simulink library "speedgoatlib_evse"  (R2024b)
settings: Solver=VariableStepAuto  StartTime=0.0  StopTime=10.0  RelTol=1e-3
undefined symbols (not defined in the file): sg_ev_charging_read_m, sg_ev_charging_write_m, sg_ev_isolation_read_m, sg_ev_parameter_read_m, sg_ev_parameter_write_m, sg_ev_precharge_read_m, sg_ev_precharge_write_m, sg_ev_status_m, sg_ev_stop_read_m, sg_ev_stop_write_m, sg_ev_welding_read_m, sg_ev_welding_write_m, sg_evse_charging_read_m, sg_evse_charging_write_m, sg_evse_isolation_read_m, sg_evse_isolation_write_m, sg_evse_parameter_read_m, sg_evse_parameter_write_m, sg_evse_precharge_read_m, sg_evse_precharge_write_m, sg_evse_status_m, sg_evse_stop_read_m, sg_evse_stop_write_m, sg_evse_welding_read_m, sg_evse_welding_write_m
libraries: speedgoatlib_mqtt x199, simulink x39, $bdroot x24
(part 7 of 8)

== system speedgoatlib_evse/Blocks by Charge State/EVSE Welding Read /Enabled Subsystem ==
  Enable : EnablePort
  ASCII to String : ASCIIToString
  ASCII to String1 : ASCIIToString
  ASCII to String2 : ASCIIToString
  Data Type Conversion1 : DataTypeConversion  OutDataTypeStr=boolean  SaturateOnIntegerOverflow=off  RndMeth=Floor
  String to Double : ScanString  Format="\"%lf\""
  String to Double1 : ScanString  Format="\"%lf\""
  String to Double2 : ScanString  Format="\"%lf\""
  port0_ci_ev_welding_errorcode : S-Function  FunctionName=sg_mqtt_client_subscribe_s  Parameters="ClientId,  ConnectionId, Topic, QoS, InitValue, Extended, SampleTime"  SFunctionDeploymentMode=off  EnableBusSupport=off  mask(mqtt_client_subscribe_1){ClientId=parClientId, ConnectionId=parConnectionId, Topic='port0/ci/ev/welding/errorcode', QoS=0 - at most once, InitValue=zeros(1,24,'uint8'), Extended=off, SampleTime=parSampleTime}
      mask prompts: ClientId "Station ID"; ConnectionId "Connection ID"; QoS "Quality of Service"; InitValue "Init Value"; Extended "Extended Interface"; SampleTime "Sample Time [s]"
      mask help: Speedgoat Driver Block<br>MQTT Client - Subscribe<br><br>&copy; 2007 - 2023, Speedgoat GmbH, <a href="matlab: web('www.speedgoat.com','-browser');">www.speedgoat.com</a>
      mask init:
      | sg_mqtt_client_subscribe_m.runMaskInitialization(ClientId, ConnectionId, Topic, InitValue, Extended);
      mask Help: eval('sg.utils.help.show(''io_main/refentry_mqtt_client_subscribe'');')
      mask TypeOptions QoS: 0 - at most once | 1 - at least once | 2 - exactly once
      mask DialogControl groupParameters Prompt: Parameters
      mask Display: disp('Speedgoat\nMQTT Client\nSubscribe\nStation ID: 0\nConnection ID: 0');
  port0_ci_ev_welding_ready : speedgoatlib_mqtt/Client/MQTT Client Subscribe  ClientId=parClientId  ConnectionId=parConnectionId  Topic='port0/ci/ev/welding/ready'  QoS=0 - at most once  InitValue=zeros(1,12,'uint8')  Extended=off  SampleTime=parSampleTime
      settings: SourceProductName=MQTT
  port0_ci_ev_welding_resssoc : S-Function  FunctionName=sg_mqtt_client_subscribe_s  Parameters="ClientId,  ConnectionId, Topic, QoS, InitValue, Extended, SampleTime"  SFunctionDeploymentMode=off  EnableBusSupport=off  mask(mqtt_client_subscribe_1){ClientId=parClientId, ConnectionId=parConnectionId, Topic='port0/ci/ev/welding/resssoc', QoS=0 - at most once, InitValue=zeros(1,12,'uint8'), Extended=off, SampleTime=parSampleTime}
      mask prompts: ClientId "Station ID"; ConnectionId "Connection ID"; QoS "Quality of Service"; InitValue "Init Value"; Extended "Extended Interface"; SampleTime "Sample Time [s]"
      mask help: Speedgoat Driver Block<br>MQTT Client - Subscribe<br><br>&copy; 2007 - 2023, Speedgoat GmbH, <a href="matlab: web('www.speedgoat.com','-browser');">www.speedgoat.com</a>
      mask init:
      | sg_mqtt_client_subscribe_m.runMaskInitialization(ClientId, ConnectionId, Topic, InitValue, Extended);
      mask Help: eval('sg.utils.help.show(''io_main/refentry_mqtt_client_subscribe'');')
      mask TypeOptions QoS: 0 - at most once | 1 - at least once | 2 - exactly once
      mask DialogControl groupParameters Prompt: Parameters
      mask Display: disp('Speedgoat\nMQTT Client\nSubscribe\nStation ID: 0\nConnection ID: 0');
  EV Ready : Outport
  EV Errorcode : Outport  Port=2
  EV RESS SOC : Outport  Port=3
  wires:
  Data Type Conversion1/1 -> EV Ready/1
  port0_ci_ev_welding_resssoc/1 -> ASCII to String2/1
  ASCII to String2/1 -> String to Double2/1
  String to Double2/1 -> EV RESS SOC/1
  String to Double1/1 -> EV Errorcode/1
  String to Double/1 -> Data Type Conversion1/1
  ASCII to String1/1 -> String to Double/1
  ASCII to String/1 -> String to Double1/1
  port0_ci_ev_welding_errorcode/1 -> ASCII to String/1
  port0_ci_ev_welding_ready/1 -> ASCII to String1/1

== system speedgoatlib_evse/Blocks by Charge State/EVSE Welding Read /string compare logic ==
  Input : Inport
  ASCII to String1 : ASCIIToString
  Add : Sum
  Gain : Gain  Gain=2
  String Compare : StringCompare
  String Compare1 : StringCompare
  String Constant : StringConstant  String="\"started\""
  String Constant1 : StringConstant  String="\"finished\""
  Out1 : Outport
  wires:
  ASCII to String1/1 -> String Compare1/1, String Compare/1
  String Constant1/1 -> String Compare1/2
  String Compare/1 -> Add/1
  String Constant/1 -> String Compare/2
  String Compare1/1 -> Gain/1
  Gain/1 -> Add/2
  Add/1 -> Out1/1
  Input/1 -> ASCII to String1/1

== system speedgoatlib_evse/Blocks by Charge State/EVSE Welding Write /Enabled Subsystem ==
  notification : Inport
  isolationstatus : Inport  Port=2
  statuscode : Inport  Port=3
  presentvoltage : Inport  Port=4
  Enable : EnablePort
  Constant1 : Constant  Value=parEnIsolationStatus  OutDataTypeStr=boolean
  Constant2 : Constant  Value=parEnStatusCode  OutDataTypeStr=boolean
  Constant3 : Constant  Value=parEnPresentVoltage  OutDataTypeStr=boolean
  Constant8 : Constant  Value=parEnNotification  OutDataTypeStr=boolean
  Data Type Conversion3 : DataTypeConversion  OutDataTypeStr=double  SaturateOnIntegerOverflow=off  RndMeth=Floor
  Data Type Conversion4 : DataTypeConversion  OutDataTypeStr=double  SaturateOnIntegerOverflow=off  RndMeth=Floor
  Function Caller11 : FunctionCaller  FunctionPrototype=json_string = toJsonPhysicalValue(multiplier,value)  InputArgumentSpecifications=double(0), double(0)  OutputArgumentSpecifications=zeros(1,48,'uint8')
  Ground{1..3,8} (4 alike) : Ground
  Simulink Function2 : Subsystem  TreatAsAtomicUnit=on
  String to ASCII1 : StringToASCII  OutputVectorSize=12
  String to ASCII2 : StringToASCII  OutputVectorSize=12
  String to ASCII3 : StringToASCII  OutputVectorSize=16
  To String1 : ToString
  To String2 : ToString
  To String3 : ToString
  port0_ci_evse_welding_isolationstatus : speedgoatlib_mqtt/Client/MQTT Client Publish  ClientId=parClientId  ConnectionId=parConnectionId  Topic='port0/ci/evse/welding/isolationstatus'  QoS=0 - at most once  Retain=on  Extended=on  SampleTime=parSampleTime
      settings: SourceProductName=MQTT
  port0_ci_evse_welding_notification : speedgoatlib_mqtt/Client/MQTT Client Publish  ClientId=parClientId  ConnectionId=parConnectionId  Topic='port0/ci/evse/welding/notification'  QoS=0 - at most once  Retain=on  Extended=on  SampleTime=parSampleTime
      settings: SourceProductName=MQTT
  port0_ci_evse_welding_presentvoltage : speedgoatlib_mqtt/Client/MQTT Client Publish  ClientId=parClientId  ConnectionId=parConnectionId  Topic='port0/ci/evse/welding/presentvoltage'  QoS=0 - at most once  Retain=on  Extended=on  SampleTime=parSampleTime
      settings: SourceProductName=MQTT
  port0_ci_evse_welding_statuscode : speedgoatlib_mqtt/Client/MQTT Client Publish  ClientId=parClientId  ConnectionId=parConnectionId  Topic='port0/ci/evse/welding/statuscode'  QoS=0 - at most once  Retain=on  Extended=on  SampleTime=parSampleTime
      settings: SourceProductName=MQTT
  to physical value format : MATLAB Function  TreatAsAtomicUnit=on
  wires:
  presentvoltage/1 -> to physical value format/1(input)
  Function Caller11/1 -> port0_ci_evse_welding_presentvoltage/1
  to physical value format/1(multiplier) -> Function Caller11/1
  to physical value format/2(value) -> Function Caller11/2
  Ground8/1 -> port0_ci_evse_welding_notification/3
  To String3/1 -> String to ASCII3/1
  Constant8/1 -> port0_ci_evse_welding_notification/2
  String to ASCII3/1 -> port0_ci_evse_welding_notification/1
  notification/1 -> To String3/1
  To String1/1 -> String to ASCII1/1
  String to ASCII1/1 -> port0_ci_evse_welding_isolationstatus/1
  Data Type Conversion3/1 -> To String1/1
  isolationstatus/1 -> Data Type Conversion3/1
  To String2/1 -> String to ASCII2/1
  statuscode/1 -> Data Type Conversion4/1
  String to ASCII2/1 -> port0_ci_evse_welding_statuscode/1
  Data Type Conversion4/1 -> To String2/1
  Constant1/1 -> port0_ci_evse_welding_isolationstatus/2
  Ground1/1 -> port0_ci_evse_welding_isolationstatus/3
  Ground2/1 -> port0_ci_evse_welding_statuscode/3
  Constant2/1 -> port0_ci_evse_welding_statuscode/2
  Constant3/1 -> port0_ci_evse_welding_presentvoltage/2
  Ground3/1 -> port0_ci_evse_welding_presentvoltage/3

== system speedgoatlib_evse/Blocks by Charge State/EVSE Welding Write /string compare logic ==
  Input : Inport
  ASCII to String1 : ASCIIToString
  Add : Sum
  Gain : Gain  Gain=2
  String Compare : StringCompare
  String Compare1 : StringCompare
  String Constant : StringConstant  String="\"started\""
  String Constant1 : StringConstant  String="\"finished\""
  Out1 : Outport
  wires:
  Input/1 -> ASCII to String1/1
  Add/1 -> Out1/1
  Gain/1 -> Add/2
  String Compare1/1 -> Gain/1
  String Constant/1 -> String Compare/2
  String Compare/1 -> Add/1
  String Constant1/1 -> String Compare1/2
  ASCII to String1/1 -> String Compare/1, String Compare1/1

== system speedgoatlib_evse/EV Status /Authentication/string compare logic ==
  Input : Inport
  ASCII to String1 : ASCIIToString
  String Compare : StringCompare  CaseSensitive=off
  String Constant : StringConstant  String="\"started\""
  Output : Outport
  wires:
  String Compare/1 -> Output/1
  String Constant/1 -> String Compare/2
  ASCII to String1/1 -> String Compare/1
  Input/1 -> ASCII to String1/1

== system speedgoatlib_evse/EV Status /Charge/string compare logic ==
  Input : Inport
  ASCII to String1 : ASCIIToString
  String Compare : StringCompare  CaseSensitive=off
  String Constant : StringConstant  String="\"started\""
  Output : Outport
  wires:
  String Constant/1 -> String Compare/2
  ASCII to String1/1 -> String Compare/1
  Input/1 -> ASCII to String1/1
  String Compare/1 -> Output/1

== system speedgoatlib_evse/EV Status /Initialization/string compare logic ==
  Input : Inport
  ASCII to String1 : ASCIIToString
  String Compare : StringCompare  CaseSensitive=off
  String Constant : StringConstant  String="\"started\""
  Output : Outport
  wires:
  ASCII to String1/1 -> String Compare/1
  String Constant/1 -> String Compare/2
  String Compare/1 -> Output/1
  Input/1 -> ASCII to String1/1

== system speedgoatlib_evse/EV Status /Isolation/string compare logic ==
  Input : Inport
  ASCII to String1 : ASCIIToString
  String Compare : StringCompare  CaseSensitive=off
  String Constant : StringConstant  String="\"started\""
  Output : Outport
  wires:
  String Constant/1 -> String Compare/2
  ASCII to String1/1 -> String Compare/1
  Input/1 -> ASCII to String1/1
  String Compare/1 -> Output/1

== system speedgoatlib_evse/EV Status /Parameter/string compare logic ==
  Input : Inport
  ASCII to String1 : ASCIIToString
  String Compare : StringCompare  CaseSensitive=off
  String Constant : StringConstant  String="\"started\""
  Output : Outport
  wires:
  String Constant/1 -> String Compare/2
  ASCII to String1/1 -> String Compare/1
  String Compare/1 -> Output/1
  Input/1 -> ASCII to String1/1

== system speedgoatlib_evse/EV Status /Precharge/string compare logic ==
  Input : Inport
  ASCII to String1 : ASCIIToString
  String Compare : StringCompare  CaseSensitive=off
  String Constant : StringConstant  String="\"started\""
  Output : Outport
  wires:
  String Constant/1 -> String Compare/2
  ASCII to String1/1 -> String Compare/1
  String Compare/1 -> Output/1
  Input/1 -> ASCII to String1/1

== system speedgoatlib_evse/EV Status /Stop/string compare logic ==
  Input : Inport
  ASCII to String1 : ASCIIToString
  String Compare : StringCompare  CaseSensitive=off
  String Constant : StringConstant  String="\"started\""
  Output : Outport
  wires:
  String Constant/1 -> String Compare/2
  ASCII to String1/1 -> String Compare/1
  Input/1 -> ASCII to String1/1
  String Compare/1 -> Output/1

== system speedgoatlib_evse/EV Status /Welding/string compare logic ==
  Input : Inport
  ASCII to String1 : ASCIIToString
  String Compare : StringCompare  CaseSensitive=off
  String Constant : StringConstant  String="\"started\""
  Output : Outport
  wires:
  String Constant/1 -> String Compare/2
  ASCII to String1/1 -> String Compare/1
  String Compare/1 -> Output/1
  Input/1 -> ASCII to String1/1

== system speedgoatlib_evse/EVSE Status /Authentication/string compare logic ==
  Input : Inport
  ASCII to String1 : ASCIIToString
  String Compare : StringCompare  CaseSensitive=off
  String Constant : StringConstant  String="\"started\""
  Output : Outport
  wires:
  Input/1 -> ASCII to String1/1
  ASCII to String1/1 -> String Compare/1
  String Constant/1 -> String Compare/2
  String Compare/1 -> Output/1

== system speedgoatlib_evse/EVSE Status /Charge/string compare logic ==
  Input : Inport
  ASCII to String1 : ASCIIToString
  String Compare : StringCompare  CaseSensitive=off
  String Constant : StringConstant  String="\"started\""
  Output : Outport
  wires:
  String Compare/1 -> Output/1
  Input/1 -> ASCII to String1/1
  ASCII to String1/1 -> String Compare/1
  String Constant/1 -> String Compare/2

== system speedgoatlib_evse/EVSE Status /Initialization/string compare logic ==
  Input : Inport
  ASCII to String1 : ASCIIToString
  String Compare : StringCompare  CaseSensitive=off
  String Constant : StringConstant  String="\"started\""
  Output : Outport
  wires:
  Input/1 -> ASCII to String1/1
  String Compare/1 -> Output/1
  String Constant/1 -> String Compare/2
  ASCII to String1/1 -> String Compare/1

== system speedgoatlib_evse/EVSE Status /Isolation/string compare logic ==
  Input : Inport
  ASCII to String1 : ASCIIToString
  String Compare : StringCompare  CaseSensitive=off
  String Constant : StringConstant  String="\"started\""
  Output : Outport
  wires:
  String Compare/1 -> Output/1
  Input/1 -> ASCII to String1/1
  ASCII to String1/1 -> String Compare/1
  String Constant/1 -> String Compare/2

== system speedgoatlib_evse/EVSE Status /Parameter/string compare logic ==
  Input : Inport
  ASCII to String1 : ASCIIToString
  String Compare : StringCompare  CaseSensitive=off
  String Constant : StringConstant  String="\"started\""
  Output : Outport
  wires:
  Input/1 -> ASCII to String1/1
  String Compare/1 -> Output/1
  ASCII to String1/1 -> String Compare/1
  String Constant/1 -> String Compare/2

== system speedgoatlib_evse/EVSE Status /Precharge/string compare logic ==
  Input : Inport
  ASCII to String1 : ASCIIToString
  String Compare : StringCompare  CaseSensitive=off
  String Constant : StringConstant  String="\"started\""
  Output : Outport
  wires:
  Input/1 -> ASCII to String1/1
  String Compare/1 -> Output/1
  ASCII to String1/1 -> String Compare/1
  String Constant/1 -> String Compare/2

== system speedgoatlib_evse/EVSE Status /Stop/string compare logic ==
  Input : Inport
  ASCII to String1 : ASCIIToString
  String Compare : StringCompare  CaseSensitive=off
  String Constant : StringConstant  String="\"started\""
  Output : Outport
  wires:
  String Compare/1 -> Output/1
  Input/1 -> ASCII to String1/1
  ASCII to String1/1 -> String Compare/1
  String Constant/1 -> String Compare/2

== system speedgoatlib_evse/EVSE Status /Welding/string compare logic ==
  Input : Inport
  ASCII to String1 : ASCIIToString
  String Compare : StringCompare  CaseSensitive=off
  String Constant : StringConstant  String="\"started\""
  Output : Outport
  wires:
  Input/1 -> ASCII to String1/1
  String Compare/1 -> Output/1
  ASCII to String1/1 -> String Compare/1
  String Constant/1 -> String Compare/2

== system speedgoatlib_evse/Blocks by Charge State/EV Charging Read /Enabled Subsystem/Simulink Function ==
  fromJsonPhysicalValue : TriggerPort  TriggerType=function-call  IsSimulinkFunction=on  FunctionName=fromJsonPhysicalValue  FunctionVisibility=scoped  VariantControl=(inherit)
  ASCII to String : ASCIIToString
  Exp : Math  Operator=10^u
  Product : Product
  Scan String : ScanString  Format='{%s %lf, %s %lf }'
  Terminator : Terminator
  Terminator1 : Terminator
  uint8_vec : ArgIn  DisableCoverage=on  OutDataTypeStr=uint8  PortDimensions=[1,48]  ArgumentName=uint8_vec
  value : ArgOut  DisableCoverage=on  ArgumentName=value
  wires:
  ASCII to String/1 -> Scan String/1
  Product/1 -> value/1
  Scan String/4 -> Product/2
  Exp/1 -> Product/1
  Scan String/2 -> Exp/1
  Scan String/3 -> Terminator1/1
  Scan String/1 -> Terminator/1
  uint8_vec/1 -> ASCII to String/1

== system speedgoatlib_evse/Blocks by Charge State/EV Charging Write /Enabled Subsystem/Simulink Function1 ==
  f : TriggerPort  TriggerType=function-call  IsSimulinkFunction=on  FunctionName=toJsonPhysicalValue  FunctionVisibility=scoped  VariantControl=(inherit)
  String Concatenate : StringConcatenate  Inputs=5
  String Constant : StringConstant  String="'{ \"Multiplier\": '"
  String Constant1 : StringConstant  String="', \"Value\": '"
  String Constant2 : StringConstant  String=' }'
  String to ASCII : StringToASCII  OutputVectorSize=48
  To String : ToString
  To String1 : ToString
  u : ArgIn  DisableCoverage=on  ArgumentName=multiplier
  u1 : ArgIn  DisableCoverage=on  Port=2  ArgumentName=value
  y : ArgOut  DisableCoverage=on  OutDataTypeStr=uint8  PortDimensions=[1,48]  ArgumentName=json_string
  wires:
  String to ASCII/1 -> y/1
  To String1/1 -> String Concatenate/4
  String Concatenate/1 -> String to ASCII/1
  To String/1 -> String Concatenate/2
  String Constant/1 -> String Concatenate/1
  u1/1 -> To String1/1
  String Constant1/1 -> String Concatenate/3
  u/1 -> To String/1
  String Constant2/1 -> String Concatenate/5

== system speedgoatlib_evse/Blocks by Charge State/EV Charging Write /Enabled Subsystem/Simulink Function2 ==
  f : TriggerPort  TriggerType=function-call  IsSimulinkFunction=on  FunctionName=toJsonPhysicalValueWithUnit  FunctionVisibility=scoped  VariantControl=(inherit)
  String Concatenate : StringConcatenate  Inputs=5
  String Constant : StringConstant  String="'{ \"Multiplier\": '"
  String Constant2 : StringConstant  String=' }'
  String Constant4 : StringConstant  String="', \"Unit\": 2, \"Value\": '"
  String to ASCII : StringToASCII  OutputVectorSize=64
  To String : ToString
  To String1 : ToString
  u : ArgIn  DisableCoverage=on  ArgumentName=multiplier
  u1 : ArgIn  DisableCoverage=on  Port=2  ArgumentName=value
  y : ArgOut  DisableCoverage=on  OutDataTypeStr=uint8  PortDimensions=[1,64]  ArgumentName=json_string
  wires:
  String to ASCII/1 -> y/1
  To String1/1 -> String Concatenate/4
  String Concatenate/1 -> String to ASCII/1
  To String/1 -> String Concatenate/2
  String Constant/1 -> String Concatenate/1
  u1/1 -> To String1/1
  String Constant4/1 -> String Concatenate/3
  u/1 -> To String/1
  String Constant2/1 -> String Concatenate/5

== system speedgoatlib_evse/Blocks by Charge State/EV Parameter Read /Enabled Subsystem/Simulink Function ==
  f : TriggerPort  TriggerType=function-call  IsSimulinkFunction=on  FunctionName=fromJsonPhysicalValue  FunctionVisibility=scoped  VariantControl=(inherit)
  ASCII to String : ASCIIToString
  Exp : Math  Operator=10^u
  Product : Product
  Scan String : ScanString  Format='{%s %lf, %s %lf }'
  Terminator : Terminator
  Terminator1 : Terminator
  uint8_vec : ArgIn  DisableCoverage=on  OutDataTypeStr=uint8  PortDimensions=[1,48]  ArgumentName=uint8_vec
  y : ArgOut  DisableCoverage=on  ArgumentName=value
  wires:
  uint8_vec/1 -> ASCII to String/1
  Scan String/1 -> Terminator/1
  Scan String/3 -> Terminator1/1
  Scan String/2 -> Exp/1
  Exp/1 -> Product/1
  Scan String/4 -> Product/2
  Product/1 -> y/1
  ASCII to String/1 -> Scan String/1

== system speedgoatlib_evse/Blocks by Charge State/EV Parameter Read /Enabled Subsystem/decode SASchedule ==
  In1 : Inport
  ASCII to String : ASCIIToString
  Power : Math  Operator=10^u
  Product : Product
  Scan String : ScanString  Format='{%s %lf, %s [ %lf ], %s [ %lf ], %s [ %lf ], %s %lf }'
  Terminator{,1..4} (5 alike) : Terminator
  SAScheduleTupleID : Outport
  SAScheduleStart : Outport  Port=2
  SAScheduelDuration : Outport  Port=3
  SASchedulePMax : Outport  Port=4
  wires:
  Scan String/2 -> SAScheduleTupleID/1
  ASCII to String/1 -> Scan String/1
  In1/1 -> ASCII to String/1
  Scan String/1 -> Terminator/1
  Scan String/3 -> Terminator1/1
  Scan String/7 -> Terminator3/1
  Scan String/5 -> Terminator2/1
  Scan String/9 -> Terminator4/1
  Power/1 -> Product/2
  Product/1 -> SASchedulePMax/1
  Scan String/4 -> Product/1
  Scan String/6 -> Power/1
  Scan String/8 -> SAScheduleStart/1
  Scan String/10 -> SAScheduelDuration/1

== system speedgoatlib_evse/Blocks by Charge State/EV Parameter Write /Enabled Subsystem/Simulink Function1 ==
  f : TriggerPort  TriggerType=function-call  IsSimulinkFunction=on  FunctionName=toJsonPhysicalValue  FunctionVisibility=scoped  VariantControl=(inherit)
  String Concatenate : StringConcatenate  Inputs=5
  String Constant : StringConstant  String="'{ \"Multiplier\": '"
  String Constant1 : StringConstant  String="', \"Value\": '"
  String Constant2 : StringConstant  String=' }'
  String to ASCII : StringToASCII  OutputVectorSize=48
  To String : ToString
  To String1 : ToString
  u : ArgIn  DisableCoverage=on  ArgumentName=multiplier
  u1 : ArgIn  DisableCoverage=on  Port=2  ArgumentName=value
  y : ArgOut  DisableCoverage=on  OutDataTypeStr=uint8  PortDimensions=[1,48]  ArgumentName=json_string
  wires:
  String Constant2/1 -> String Concatenate/5
  u/1 -> To String/1
  String Constant1/1 -> String Concatenate/3
  u1/1 -> To String1/1
  String Constant/1 -> String Concatenate/1
  To String/1 -> String Concatenate/2
  String Concatenate/1 -> String to ASCII/1
  To String1/1 -> String Concatenate/4
  String to ASCII/1 -> y/1

== system speedgoatlib_evse/Blocks by Charge State/EV Pre-Charge Read /Enabled Subsystem/Simulink Function ==
  fromJsonPhysicalValue : TriggerPort  TriggerType=function-call  IsSimulinkFunction=on  FunctionName=fromJsonPhysicalValue  FunctionVisibility=scoped  VariantControl=(inherit)
  ASCII to String : ASCIIToString
  Exp : Math  Operator=10^u
  Product : Product
  Scan String : ScanString  Format='{%s %lf, %s %lf }'
  Terminator : Terminator
  Terminator1 : Terminator
  uint8_vec : ArgIn  DisableCoverage=on  OutDataTypeStr=uint8  PortDimensions=[1,48]  ArgumentName=uint8_vec
  value : ArgOut  DisableCoverage=on  ArgumentName=value
  wires:
  ASCII to String/1 -> Scan String/1
  Product/1 -> value/1
  Scan String/4 -> Product/2
  Exp/1 -> Product/1
  Scan String/2 -> Exp/1
  Scan String/3 -> Terminator1/1
  Scan String/1 -> Terminator/1
  uint8_vec/1 -> ASCII to String/1

== system speedgoatlib_evse/Blocks by Charge State/EV Pre-Charge Write /Enabled Subsystem/Simulink Function1 ==
  f : TriggerPort  TriggerType=function-call  IsSimulinkFunction=on  FunctionName=toJsonPhysicalValue  FunctionVisibility=scoped  VariantControl=(inherit)
  String Concatenate : StringConcatenate  Inputs=5
  String Constant : StringConstant  String="'{ \"Multiplier\": '"
  String Constant1 : StringConstant  String="', \"Value\": '"
  String Constant2 : StringConstant  String=' }'
  String to ASCII : StringToASCII  OutputVectorSize=48
  To String : ToString
  To String1 : ToString
  u : ArgIn  DisableCoverage=on  ArgumentName=multiplier
  u1 : ArgIn  DisableCoverage=on  Port=2  ArgumentName=value
  y : ArgOut  DisableCoverage=on  OutDataTypeStr=uint8  PortDimensions=[1,48]  ArgumentName=json_string
  wires:
  String to ASCII/1 -> y/1
  To String1/1 -> String Concatenate/4
  String Concatenate/1 -> String to ASCII/1
  To String/1 -> String Concatenate/2
  String Constant/1 -> String Concatenate/1
  u1/1 -> To String1/1
  String Constant1/1 -> String Concatenate/3
  u/1 -> To String/1
  String Constant2/1 -> String Concatenate/5

== system speedgoatlib_evse/Blocks by Charge State/EV Setup /Enabled Subsystem/Simulink Function ==
  f : TriggerPort  TriggerType=function-call  IsSimulinkFunction=on  FunctionName=toJsonPhysicalValue  FunctionVisibility=scoped  VariantControl=(inherit)
  String Concatenate : StringConcatenate  Inputs=5
  String Constant : StringConstant  String="'{ \"Multiplier\": '"
  String Constant1 : StringConstant  String="', \"Value\": '"
  String Constant2 : StringConstant  String=' }'
  String to ASCII : StringToASCII  OutputVectorSize=48
  To String : ToString
  To String1 : ToString
  u : ArgIn  DisableCoverage=on  ArgumentName=multiplier
  u1 : ArgIn  DisableCoverage=on  Port=2  ArgumentName=value
  y : ArgOut  DisableCoverage=on  OutDataTypeStr=uint8  PortDimensions=[1,48]  ArgumentName=json_string
  wires:
  String Constant2/1 -> String Concatenate/5
  u/1 -> To String/1
  String Constant1/1 -> String Concatenate/3
  u1/1 -> To String1/1
  String Constant/1 -> String Concatenate/1
  To String/1 -> String Concatenate/2
  String Concatenate/1 -> String to ASCII/1
  To String1/1 -> String Concatenate/4
  String to ASCII/1 -> y/1

== system speedgoatlib_evse/Blocks by Charge State/EV Welding Read /Enabled Subsystem/Simulink Function ==
  fromJsonPhysicalValue : TriggerPort  TriggerType=function-call  IsSimulinkFunction=on  FunctionName=fromJsonPhysicalValue  FunctionVisibility=scoped  VariantControl=(inherit)
  ASCII to String : ASCIIToString
  Exp : Math  Operator=10^u
  Product : Product
  Scan String : ScanString  Format='{%s %lf, %s %lf }'
  Terminator : Terminator
  Terminator1 : Terminator
  uint8_vec : ArgIn  DisableCoverage=on  OutDataTypeStr=uint8  PortDimensions=[1,48]  ArgumentName=uint8_vec
  value : ArgOut  DisableCoverage=on  ArgumentName=value
  wires:
  uint8_vec/1 -> ASCII to String/1
  Scan String/1 -> Terminator/1
  Scan String/3 -> Terminator1/1
  Scan String/2 -> Exp/1
  Exp/1 -> Product/1
  Scan String/4 -> Product/2
  Product/1 -> value/1
  ASCII to String/1 -> Scan String/1

== system speedgoatlib_evse/Blocks by Charge State/EVSE Charging Read /Enabled Subsystem/Simulink Function ==
  f : TriggerPort  TriggerType=function-call  IsSimulinkFunction=on  FunctionName=fromJsonPhysicalValue  FunctionVisibility=scoped  VariantControl=(inherit)
  ASCII to String : ASCIIToString
  Exp : Math  Operator=10^u
  Product : Product
  Scan String : ScanString  Format='{%s %lf, %s %lf }'
  Terminator : Terminator
  Terminator1 : Terminator
  uint8_vec : ArgIn  DisableCoverage=on  OutDataTypeStr=uint8  PortDimensions=[1,48]  ArgumentName=uint8_vec
  y : ArgOut  DisableCoverage=on  ArgumentName=value
  wires:
  uint8_vec/1 -> ASCII to String/1
  Scan String/1 -> Terminator/1
  Scan String/3 -> Terminator1/1
  Scan String/2 -> Exp/1
  Exp/1 -> Product/1
  Scan String/4 -> Product/2
  Product/1 -> y/1
  ASCII to String/1 -> Scan String/1

== system speedgoatlib_evse/Blocks by Charge State/EVSE Charging Read /Enabled Subsystem/Simulink Function1 ==
  f : TriggerPort  TriggerType=function-call  IsSimulinkFunction=on  FunctionName=fromJsonPhysicalValueUnit  FunctionVisibility=scoped  VariantControl=(inherit)
  ASCII to String : ASCIIToString
  Exp : Math  Operator=10^u
  Hours : Subsystem  TreatAsAtomicUnit=on
  Merge : Merge  Inputs=3
  Minutes : Subsystem  TreatAsAtomicUnit=on
  Product : Product
  Product1 : Product
  Scan String : ScanString  Format='{%s %lf, %s %lf, %s %lf }'
  Seconds : Subsystem  TreatAsAtomicUnit=on
  Switch Case : SwitchCase  CaseConditions={0, 1, 2}  ShowDefaultCase=off
  Terminator : Terminator
  Terminator1 : Terminator
  Terminator2 : Terminator
  uint8_vec : ArgIn  DisableCoverage=on  OutDataTypeStr=uint8  PortDimensions=[1,64]  ArgumentName=uint8_vec
  y : ArgOut  DisableCoverage=on  ArgumentName=value
  wires:
  ASCII to String/1 -> Scan String/1
  Product/1 -> Product1/1
  Scan String/6 -> Product/2
  Exp/1 -> Product/1
  Scan String/2 -> Exp/1
  Scan String/3 -> Terminator1/1
  Scan String/1 -> Terminator/1
  uint8_vec/1 -> ASCII to String/1
  Scan String/5 -> Terminator2/1
  Scan String/4 -> Switch Case/1
  Switch Case/1 -> Hours/Action
  Switch Case/2 -> Minutes/Action
  Switch Case/3 -> Seconds/Action
  Hours/1(Out1) -> Merge/1
  Minutes/1(Out1) -> Merge/2
  Seconds/1(Out1) -> Merge/3
  Merge/1 -> Product1/2
  Product1/1 -> y/1

== system speedgoatlib_evse/Blocks by Charge State/EVSE Charging Write /Enabled Subsystem/Simulink Function2 ==
  f : TriggerPort  TriggerType=function-call  IsSimulinkFunction=on  FunctionName=toJsonPhysicalValue  FunctionVisibility=scoped  VariantControl=(inherit)
  String Concatenate : StringConcatenate  Inputs=5
  String Constant : StringConstant  String="'{ \"Multiplier\": '"
  String Constant1 : StringConstant  String="', \"Value\": '"
  String Constant2 : StringConstant  String=' }'
  String to ASCII : StringToASCII  OutputVectorSize=48
  To String : ToString
  To String1 : ToString
  u : ArgIn  DisableCoverage=on  ArgumentName=multiplier
  u1 : ArgIn  DisableCoverage=on  Port=2  ArgumentName=value
  y : ArgOut  DisableCoverage=on  OutDataTypeStr=uint8  PortDimensions=[1,48]  ArgumentName=json_string
  wires:
  String to ASCII/1 -> y/1
  To String1/1 -> String Concatenate/4
  String Concatenate/1 -> String to ASCII/1
  To String/1 -> String Concatenate/2
  String Constant/1 -> String Concatenate/1
  u1/1 -> To String1/1
  String Constant1/1 -> String Concatenate/3
  u/1 -> To String/1
  String Constant2/1 -> String Concatenate/5

== system speedgoatlib_evse/Blocks by Charge State/EVSE Parameter Read /Enabled Subsystem/Simulink Function ==
  f : TriggerPort  TriggerType=function-call  IsSimulinkFunction=on  FunctionName=fromJsonPhysicalValue  FunctionVisibility=scoped  VariantControl=(inherit)
  ASCII to String : ASCIIToString
  Exp : Math  Operator=10^u
  Product : Product
  Scan String : ScanString  Format='{%s %lf, %s %lf }'
  Terminator : Terminator
  Terminator1 : Terminator
  uint8_vec : ArgIn  DisableCoverage=on  OutDataTypeStr=uint8  PortDimensions=[1,48]  ArgumentName=uint8_vec
  y : ArgOut  DisableCoverage=on  ArgumentName=value
  wires:
  ASCII to String/1 -> Scan String/1
  Product/1 -> y/1
  Scan String/4 -> Product/2
  Exp/1 -> Product/1
  Scan String/2 -> Exp/1
  Scan String/3 -> Terminator1/1
  Scan String/1 -> Terminator/1
  uint8_vec/1 -> ASCII to String/1

== system speedgoatlib_evse/Blocks by Charge State/EVSE Parameter Write /Enabled Subsystem/Simulink Function1 ==
  f : TriggerPort  TriggerType=function-call  IsSimulinkFunction=on  FunctionName=toJsonPhysicalValue  FunctionVisibility=scoped  VariantControl=(inherit)
  String Concatenate : StringConcatenate  Inputs=5
  String Constant : StringConstant  String="'{ \"Multiplier\": '"
  String Constant1 : StringConstant  String="', \"Value\": '"
  String Constant2 : StringConstant  String=' }'
  String to ASCII : StringToASCII  OutputVectorSize=48
  To String : ToString
  To String1 : ToString
  u : ArgIn  DisableCoverage=on  ArgumentName=multiplier
  u1 : ArgIn  DisableCoverage=on  Port=2  ArgumentName=value
  y : ArgOut  DisableCoverage=on  OutDataTypeStr=uint8  PortDimensions=[1,48]  ArgumentName=json_string
  wires:
  String Constant2/1 -> String Concatenate/5
  u/1 -> To String/1
  String Constant1/1 -> String Concatenate/3
  u1/1 -> To String1/1
  String Constant/1 -> String Concatenate/1
  To String/1 -> String Concatenate/2
  String Concatenate/1 -> String to ASCII/1
  To String1/1 -> String Concatenate/4
  String to ASCII/1 -> y/1

== system speedgoatlib_evse/Blocks by Charge State/EVSE Parameter Write /Enabled Subsystem/to SASchedule JSON ==
  ID : Inport
  Start : Inport  Port=2
  Duration : Inport  Port=3
  PMaxMult : Inport  Port=4
  PMax : Inport  Port=5
  String Concatenate : StringConcatenate  Inputs=11
  String Constant : StringConstant  String="'{ \"SAScheduleTupleID\" : '"
  String Constant1 : StringConstant  String="', \"Start\" : ['"
  String Constant2 : StringConstant  String="'], \"Duration\" : '"
  String Constant3 : StringConstant  String="', \"PMax\" : ['"
  String Constant4 : StringConstant  String="'], \"PMaxMultiplier\" : ['"
  String Constant5 : StringConstant  String='] }'
  String to ASCII : StringToASCII  OutputVectorSize=255
  To String{,1..4} (5 alike) : ToString
  JSON string output : Outport
  wires:
  To String4/1 -> String Concatenate/10
  To String3/1 -> String Concatenate/8
  To String2/1 -> String Concatenate/6
  Duration/1 -> To String2/1
  String Constant3/1 -> String Concatenate/7
  PMax/1 -> To String3/1
  String Constant4/1 -> String Concatenate/9
  PMaxMult/1 -> To String4/1
  String Constant5/1 -> String Concatenate/11
  Start/1 -> To String1/1
  String Constant2/1 -> String Concatenate/5
  To String1/1 -> String Concatenate/4
  ID/1 -> To String/1
  To String/1 -> String Concatenate/2
  String Concatenate/1 -> String to ASCII/1
  String Constant/1 -> String Concatenate/1
  String Constant1/1 -> String Concatenate/3
  String to ASCII/1 -> JSON string output/1

== system speedgoatlib_evse/Blocks by Charge State/EVSE Pre-Charge Read /Enabled Subsystem/Simulink Function ==
  f : TriggerPort  TriggerType=function-call  IsSimulinkFunction=on  FunctionName=fromJsonPhysicalValue  FunctionVisibility=scoped  VariantControl=(inherit)
  ASCII to String : ASCIIToString
  Exp : Math  Operator=10^u
  Product : Product
  Scan String : ScanString  Format='{%s %lf, %s %lf }'
  Terminator : Terminator
  Terminator1 : Terminator
  uint8_vec : ArgIn  DisableCoverage=on  OutDataTypeStr=uint8  PortDimensions=[1,48]  ArgumentName=uint8_vec
  y : ArgOut  DisableCoverage=on  ArgumentName=value
  wires:
  uint8_vec/1 -> ASCII to String/1
  Scan String/1 -> Terminator/1
  Scan String/3 -> Terminator1/1
  Scan String/2 -> Exp/1
  Exp/1 -> Product/1
  Scan String/4 -> Product/2
  Product/1 -> y/1
  ASCII to String/1 -> Scan String/1

== system speedgoatlib_evse/Blocks by Charge State/EVSE Pre-Charge Write /Enabled Subsystem/Simulink Function2 ==
  f : TriggerPort  TriggerType=function-call  IsSimulinkFunction=on  FunctionName=toJsonPhysicalValue  FunctionVisibility=scoped  VariantControl=(inherit)
  String Concatenate : StringConcatenate  Inputs=5
  String Constant : StringConstant  String="'{ \"Multiplier\": '"
  String Constant1 : StringConstant  String="', \"Value\": '"
  String Constant2 : StringConstant  String=' }'
  String to ASCII : StringToASCII  OutputVectorSize=48
  To String : ToString
  To String1 : ToString
  u : ArgIn  DisableCoverage=on  ArgumentName=multiplier
  u1 : ArgIn  DisableCoverage=on  Port=2  ArgumentName=value
  y : ArgOut  DisableCoverage=on  OutDataTypeStr=uint8  PortDimensions=[1,48]  ArgumentName=json_string
  wires:
  String to ASCII/1 -> y/1
  To String1/1 -> String Concatenate/4
  String Concatenate/1 -> String to ASCII/1
  To String/1 -> String Concatenate/2
  String Constant/1 -> String Concatenate/1
  u1/1 -> To String1/1
  String Constant1/1 -> String Concatenate/3
  u/1 -> To String/1
  String Constant2/1 -> String Concatenate/5

== system speedgoatlib_evse/Blocks by Charge State/EVSE Setup /Enabled Subsystem/Simulink Function ==
  f : TriggerPort  TriggerType=function-call  IsSimulinkFunction=on  FunctionName=toJsonPhysicalValue  FunctionVisibility=scoped  VariantControl=(inherit)
  String Concatenate : StringConcatenate  Inputs=5
  String Constant : StringConstant  String="'{ \"Multiplier\": '"
  String Constant1 : StringConstant  String="', \"Value\": '"
  String Constant2 : StringConstant  String=' }'
  String to ASCII : StringToASCII  OutputVectorSize=48
  To String : ToString
  To String1 : ToString
  u : ArgIn  DisableCoverage=on  ArgumentName=multiplier
  u1 : ArgIn  DisableCoverage=on  Port=2  ArgumentName=value
  y : ArgOut  DisableCoverage=on  OutDataTypeStr=uint8  PortDimensions=[1,48]  ArgumentName=json_string
  wires:
  String to ASCII/1 -> y/1
  To String1/1 -> String Concatenate/4
  String Concatenate/1 -> String to ASCII/1
  To String/1 -> String Concatenate/2
  String Constant/1 -> String Concatenate/1
  u1/1 -> To String1/1
  String Constant1/1 -> String Concatenate/3
  u/1 -> To String/1
  String Constant2/1 -> String Concatenate/5

== system speedgoatlib_evse/Blocks by Charge State/EVSE Welding Write /Enabled Subsystem/Simulink Function2 ==
  f : TriggerPort  TriggerType=function-call  IsSimulinkFunction=on  FunctionName=toJsonPhysicalValue  FunctionVisibility=scoped  VariantControl=(inherit)
  String Concatenate : StringConcatenate  Inputs=5
  String Constant : StringConstant  String="'{ \"Multiplier\": '"
  String Constant1 : StringConstant  String="', \"Value\": '"
  String Constant2 : StringConstant  String=' }'
  String to ASCII : StringToASCII  OutputVectorSize=48
  To String : ToString
  To String1 : ToString
  u : ArgIn  DisableCoverage=on  ArgumentName=multiplier
  u1 : ArgIn  DisableCoverage=on  Port=2  ArgumentName=value
  y : ArgOut  DisableCoverage=on  OutDataTypeStr=uint8  PortDimensions=[1,48]  ArgumentName=json_string
  wires:
  String Constant2/1 -> String Concatenate/5
  u/1 -> To String/1
  String Constant1/1 -> String Concatenate/3
  u1/1 -> To String1/1
  String Constant/1 -> String Concatenate/1
  To String/1 -> String Concatenate/2
  String Concatenate/1 -> String to ASCII/1
  To String1/1 -> String Concatenate/4
  String to ASCII/1 -> y/1

== system speedgoatlib_evse/Blocks by Charge State/EVSE Charging Read /Enabled Subsystem/Simulink Function1/Hours ==
  Action Port : ActionPort
  Constant : Constant  Value=3600
  Out1 : Outport  InitialOutput=3600
  wires:
  Constant/1 -> Out1/1

== system speedgoatlib_evse/Blocks by Charge State/EVSE Charging Read /Enabled Subsystem/Simulink Function1/Minutes ==
  Action Port : ActionPort
  Constant : Constant  Value=60
  Out1 : Outport  InitialOutput=60
  wires:
  Constant/1 -> Out1/1

== system speedgoatlib_evse/Blocks by Charge State/EVSE Charging Read /Enabled Subsystem/Simulink Function1/Seconds ==
  Action Port : ActionPort
  Constant : Constant
  Out1 : Outport  InitialOutput=1
  wires:
  Constant/1 -> Out1/1

== matlab function speedgoatlib_evse/Blocks by Charge State/EV Charging Write /Enabled Subsystem/to physical value format1 ==
  data: multiplier output; input input; value output
function [multiplier, value] = fcn(input)
    [multiplier, value] = sg_evse.lib_m.toJsonPhysicalValue(input);
end

== matlab function speedgoatlib_evse/Blocks by Charge State/EVSE Setup /Enabled Subsystem/to physical value format6 ==
  data: multiplier output; input input; value output
function [multiplier, value] = fcn(input)
    [multiplier, value] = sg_evse.lib_m.toJsonPhysicalValue(input);
end

== matlab function speedgoatlib_evse/Blocks by Charge State/EVSE Setup /Enabled Subsystem/to physical value format7 ==
  data: multiplier output; input input; value output
function [multiplier, value] = fcn(input)
    [multiplier, value] = sg_evse.lib_m.toJsonPhysicalValue(input);
end

== matlab function speedgoatlib_evse/Blocks by Charge State/EVSE Setup /Enabled Subsystem/to physical value format8 ==
  data: multiplier output; input input; value output
function [multiplier, value] = fcn(input)
    [multiplier, value] = sg_evse.lib_m.toJsonPhysicalValue(input);
end

== matlab function speedgoatlib_evse/Blocks by Charge State/EVSE Setup /Enabled Subsystem/to physical value format9 ==
  data: multiplier output; input input; value output
function [multiplier, value] = fcn(input)
    [multiplier, value] = sg_evse.lib_m.toJsonPhysicalValue(input);
end

== matlab function speedgoatlib_evse/Blocks by Charge State/EV Setup /Enabled Subsystem/to physical value format1 ==
  data: multiplier output; input input; value output
function [multiplier, value] = fcn(input)
    [multiplier, value] = sg_evse.lib_m.toJsonPhysicalValue(input);
end

== matlab function speedgoatlib_evse/Blocks by Charge State/EV Parameter Write /Enabled Subsystem/to physical value format1 ==
  data: multiplier output; input input; value output
function [multiplier, value] = fcn(input)
    [multiplier, value] = sg_evse.lib_m.toJsonPhysicalValue(input);
end

== matlab function speedgoatlib_evse/Blocks by Charge State/EV Parameter Write /Enabled Subsystem/to physical value format2 ==
  data: multiplier output; input input; value output
function [multiplier, value] = fcn(input)
    [multiplier, value] = sg_evse.lib_m.toJsonPhysicalValue(input);
end

== matlab function speedgoatlib_evse/Blocks by Charge State/EV Charging Write /Enabled Subsystem/to physical value format2 ==
  data: multiplier output; input input; value output
function [multiplier, value] = fcn(input)
    [multiplier, value] = sg_evse.lib_m.toJsonPhysicalValue(input);
end

== matlab function speedgoatlib_evse/Blocks by Charge State/EV Charging Write /Enabled Subsystem/to physical value format3 ==
  data: multiplier output; input input; value output
function [multiplier, value] = fcn(input)
    [multiplier, value] = sg_evse.lib_m.toJsonPhysicalValue(input);
end

== matlab function speedgoatlib_evse/Blocks by Charge State/EV Pre-Charge Write /Enabled Subsystem/to physical value format ==
  data: multiplier output; input input; value output
function [multiplier, value] = fcn(input)
    [multiplier, value] = sg_evse.lib_m.toJsonPhysicalValue(input);
end

== matlab function speedgoatlib_evse/Blocks by Charge State/EV Pre-Charge Write /Enabled Subsystem/to physical value format1 ==
  data: multiplier output; input input; value output
function [multiplier, value] = fcn(input)
    [multiplier, value] = sg_evse.lib_m.toJsonPhysicalValue(input);
end

== matlab function speedgoatlib_evse/Blocks by Charge State/EVSE Pre-Charge Write /Enabled Subsystem/to physical value format ==
  data: multiplier output; input input; value output
function [multiplier, value] = fcn(input)
    [multiplier, value] = sg_evse.lib_m.toJsonPhysicalValue(input);
end

== matlab function speedgoatlib_evse/Blocks by Charge State/EVSE Welding Write /Enabled Subsystem/to physical value format ==
  data: multiplier output; input input; value output
function [multiplier, value] = fcn(input)
    [multiplier, value] = sg_evse.lib_m.toJsonPhysicalValue(input);
end

== matlab function speedgoatlib_evse/EVSE Status /MATLAB Function ==
  data: u1 input; y output; u2 input; u3 input; u4 input; u5 input; u6 input; u7 input; u8 input
function y = fcn(u1, u2, u3, u4, u5, u6, u7, u8)
    u = [u1 u2 u3 u4 u5 u6 u7 u8];
    y = min(u(u>0));
end

== matlab function speedgoatlib_evse/Blocks by Charge State/EV Setup /Enabled Subsystem/to physical value format ==
  data: multiplier output; input input; value output
function [multiplier, value] = fcn(input)
    [multiplier, value] = sg_evse.lib_m.toJsonPhysicalValue(input);
end

== matlab function speedgoatlib_evse/EV Status /MATLAB Function ==
  data: u1 input; y output; u2 input; u3 input; u4 input; u5 input; u6 input; u7 input; u8 input
function y = fcn(u1, u2, u3, u4, u5, u6, u7, u8)
    u = [u1 u2 u3 u4 u5 u6 u7 u8];
    y = min(u(u>0));
end

== matlab function speedgoatlib_evse/Blocks by Charge State/EV Parameter Write /Enabled Subsystem/to physical value format3 ==
  data: multiplier output; input input; value output
function [multiplier, value] = fcn(input)
    [multiplier, value] = sg_evse.lib_m.toJsonPhysicalValue(input);
end

== matlab function speedgoatlib_evse/Blocks by Charge State/EV Parameter Write /Enabled Subsystem/to physical value format7 ==
  data: multiplier output; input input; value output
function [multiplier, value] = fcn(input)
    [multiplier, value] = sg_evse.lib_m.toJsonPhysicalValue(input);
end

== matlab function speedgoatlib_evse/Blocks by Charge State/EV Parameter Write /Enabled Subsystem/to physical value format8 ==
  data: multiplier output; input input; value output
function [multiplier, value] = fcn(input)
    [multiplier, value] = sg_evse.lib_m.toJsonPhysicalValue(input);
end

== matlab function speedgoatlib_evse/Blocks by Charge State/EV Parameter Write /Enabled Subsystem/to physical value format9 ==
  data: multiplier output; input input; value output
function [multiplier, value] = fcn(input)
    [multiplier, value] = sg_evse.lib_m.toJsonPhysicalValue(input);
end

== matlab function speedgoatlib_evse/Blocks by Charge State/EVSE Charging Write /Enabled Subsystem/to physical value format ==
  data: multiplier output; input input; value output
function [multiplier, value] = fcn(input)
    [multiplier, value] = sg_evse.lib_m.toJsonPhysicalValue(input);
end

== matlab function speedgoatlib_evse/Blocks by Charge State/EVSE Charging Write /Enabled Subsystem/to physical value format1 ==
  data: multiplier output; input input; value output
function [multiplier, value] = fcn(input)
    [multiplier, value] = sg_evse.lib_m.toJsonPhysicalValue(input);
end

== matlab function speedgoatlib_evse/Blocks by Charge State/EVSE Charging Write /Enabled Subsystem/to physical value format7 ==
  data: multiplier output; input input; value output
function [multiplier, value] = fcn(input)
    [multiplier, value] = sg_evse.lib_m.toJsonPhysicalValue(input);
end

== matlab function speedgoatlib_evse/Blocks by Charge State/EVSE Charging Write /Enabled Subsystem/to physical value format8 ==
  data: multiplier output; input input; value output
function [multiplier, value] = fcn(input)
    [multiplier, value] = sg_evse.lib_m.toJsonPhysicalValue(input);
end

== matlab function speedgoatlib_evse/Blocks by Charge State/EVSE Charging Write /Enabled Subsystem/to physical value format9 ==
  data: multiplier output; input input; value output
function [multiplier, value] = fcn(input)
    [multiplier, value] = sg_evse.lib_m.toJsonPhysicalValue(input);
end

== matlab function speedgoatlib_evse/Blocks by Charge State/EV Setup /Enabled Subsystem/to physical value format2 ==
  data: multiplier output; input input; value output
function [multiplier, value] = fcn(input)
    [multiplier, value] = sg_evse.lib_m.toJsonPhysicalValue(input);
end

== matlab function speedgoatlib_evse/Blocks by Charge State/EVSE Parameter Write /Enabled Subsystem/to physical value format1 ==
  data: multiplier output; input input; value output
function [multiplier, value] = fcn(input)
    [multiplier, value] = sg_evse.lib_m.toJsonPhysicalValue(input);
end

== matlab function speedgoatlib_evse/Blocks by Charge State/EVSE Parameter Write /Enabled Subsystem/to physical value format2 ==
  data: multiplier output; input input; value output
function [multiplier, value] = fcn(input)
    [multiplier, value] = sg_evse.lib_m.toJsonPhysicalValue(input);
end

== matlab function speedgoatlib_evse/Blocks by Charge State/EVSE Parameter Write /Enabled Subsystem/to physical value format3 ==
  data: multiplier output; input input; value output
function [multiplier, value] = fcn(input)
    [multiplier, value] = sg_evse.lib_m.toJsonPhysicalValue(input);
end

== matlab function speedgoatlib_evse/Blocks by Charge State/EVSE Parameter Write /Enabled Subsystem/to physical value format4 ==
  data: multiplier output; input input; value output
function [multiplier, value] = fcn(input)
    [multiplier, value] = sg_evse.lib_m.toJsonPhysicalValue(input);
end

== matlab function speedgoatlib_evse/Blocks by Charge State/EVSE Parameter Write /Enabled Subsystem/to physical value format5 ==
  data: multiplier output; input input; value output
function [multiplier, value] = fcn(input)
    [multiplier, value] = sg_evse.lib_m.toJsonPhysicalValue(input);
end

== matlab function speedgoatlib_evse/Blocks by Charge State/EVSE Parameter Write /Enabled Subsystem/to physical value format6 ==
  data: multiplier output; input input; value output
function [multiplier, value] = fcn(input)
    [multiplier, value] = sg_evse.lib_m.toJsonPhysicalValue(input);
end

== matlab function speedgoatlib_evse/Blocks by Charge State/EVSE Parameter Write /Enabled Subsystem/to physical value format7 ==
  data: multiplier output; input input; value output
function [multiplier, value] = fcn(input)
    [multiplier, value] = sg_evse.lib_m.toJsonPhysicalValue(input);
end

== matlab function speedgoatlib_evse/Blocks by Charge State/EVSE Parameter Write /Enabled Subsystem/to physical value format8 ==
  data: multiplier output; input input; value output
function [multiplier, value] = fcn(input)
    [multiplier, value] = sg_evse.lib_m.toJsonPhysicalValue(input);
end

== matlab function speedgoatlib_evse/Blocks by Charge State/EVSE Parameter Write /Enabled Subsystem/to physical value format9 ==
  data: multiplier output; input input; value output
function [multiplier, value] = fcn(input)
    [multiplier, value] = sg_evse.lib_m.toJsonPhysicalValue(input);
end

== matlab function speedgoatlib_evse/Blocks by Charge State/EV Setup /Enabled Subsystem/to physical value format3 ==
  data: multiplier output; input input; value output
function [multiplier, value] = fcn(input)
    [multiplier, value] = sg_evse.lib_m.toJsonPhysicalValue(input);
end

== matlab function speedgoatlib_evse/Blocks by Charge State/EV Setup /Enabled Subsystem/to physical value format4 ==
  data: multiplier output; input input; value output
function [multiplier, value] = fcn(input)
    [multiplier, value] = sg_evse.lib_m.toJsonPhysicalValue(input);
end

== matlab function speedgoatlib_evse/Blocks by Charge State/EV Setup /Enabled Subsystem/to physical value format5 ==
  data: multiplier output; input input; value output
function [multiplier, value] = fcn(input)
    [multiplier, value] = sg_evse.lib_m.toJsonPhysicalValue(input);
end
